simulink library "rpm_2_torque_lib"  (R2018b)
settings: Solver=VariableStepAuto  StartTime=0.0  StopTime=10.0  RelTol=1e-3
undefined symbols (not defined in the file or in its folder): simParams
settings Model: Creator=Taylor  LastModifiedBy=Taylor

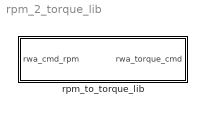
== system rpm_2_torque_lib ==
  rpm_to_torque_lib : Subsystem

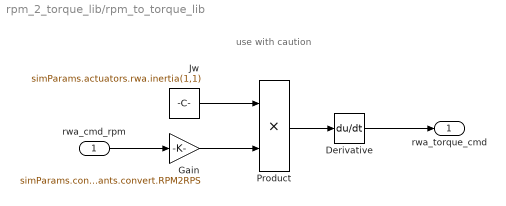
== system rpm_2_torque_lib/rpm_to_torque_lib ==
  note: use with caution
  rwa_cmd_rpm : Inport
  Derivative : Derivative
  Gain : Gain  Gain=simParams.constants.convert.RPM2RPS
  Jw : Constant  Value=simParams.actuators.rwa.inertia(1,1)
  Product : Product
  rwa_torque_cmd : Outport
  wires:
  rwa_cmd_rpm/1 -> Gain/1
  Jw/1 -> Product/1
  Product/1 -> Derivative/1
  Gain/1 -> Product/2
  Derivative/1 -> rwa_torque_cmd/1
